simulink model "buffer_delay1"  (Simulink 5.1)
settings: Solver=ode45  StartTime=0.0  StopTime=30.0  RelTol=1e-3
libraries: dspbuff3 x5, dspsigattribs x3, dspindex x1, simulink x1
settings Model: Creator=svenhoffmann  LastModifiedBy=svenhoffmann  ExtModeAutoUpdateStatusClock=off  BooleanDataType=on  ProdHWDeviceType=Microprocessor

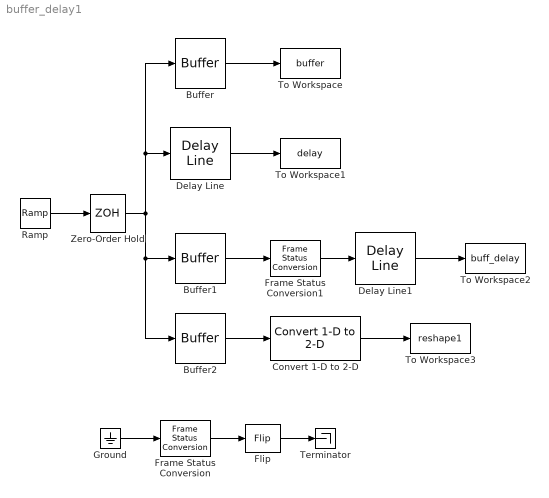
== system buffer_delay1 ==
  Buffer : dspbuff3/Buffer  N=5  V=0  ic=0
  Buffer1 : dspbuff3/Buffer  N=5  V=0  ic=0
  Buffer2 : dspbuff3/Buffer  N=50  V=45  ic=0
  Convert 1-D to 2-D : dspsigattribs/Convert 1-D to 2-D  M=5  N=10  frameBasedOut=off
  Delay Line : dspbuff3/Delay Line  siz=5  ic=0  directfeed=off
  Delay Line1 : dspbuff3/Delay Line  siz=10  ic=0  directfeed=on
  Flip : dspindex/Flip  dim=Columns
  Frame Status Conversion : dspsigattribs/Frame Status Conversion  growRefPort=off  outframe=Frame-based
  Frame Status Conversion1 : dspsigattribs/Frame Status Conversion  growRefPort=off  outframe=Sample-based
  Ground : Ground
  Ramp : simulink/Sources/Ramp  slope=1  start=0  X0=0
  Terminator : Terminator
  To Workspace : ToWorkspace  VariableName=buffer  SampleTime=1  SaveFormat=Array
  To Workspace1 : ToWorkspace  VariableName=delay  SampleTime=1  SaveFormat=Array
  To Workspace2 : ToWorkspace  VariableName=buff_delay  SampleTime=1  SaveFormat=Array
  To Workspace3 : ToWorkspace  VariableName=reshape1  SampleTime=1  SaveFormat=Array
  Zero-Order Hold : ZeroOrderHold
  wires:
  Ramp/1 -> Zero-Order Hold/1
  Zero-Order Hold/1 -> Buffer/1, Delay Line/1, Buffer1/1, Buffer2/1
  Buffer1/1 -> Frame Status Conversion1/1
  Buffer/1 -> To Workspace/1
  Delay Line/1 -> To Workspace1/1
  Delay Line1/1 -> To Workspace2/1
  Ground/1 -> Frame Status Conversion/1
  Frame Status Conversion/1 -> Flip/1
  Flip/1 -> Terminator/1
  Convert 1-D to 2-D/1 -> To Workspace3/1
  Buffer2/1 -> Convert 1-D to 2-D/1
  Frame Status Conversion1/1 -> Delay Line1/1
